simulink model "GA_PID_2DOF"  (R2024b)
settings: Solver=VariableStepDiscrete  StartTime=0.0  StopTime=40  RelTol=1e-3
values from neighbouring files (symbols this model uses):
  Kd1 = par(bestchrom, 3)    [GA_PID_Main.m]    (also in main_GA.m = par(pop_index, 3))
  Kd2 = par(bestchrom, 6)    [GA_PID_Main.m]    (also in main_GA.m = par(pop_index, 6))
  Ki1 = par(bestchrom, 2)    [GA_PID_Main.m]    (also in main_GA.m = par(pop_index, 2))
  Ki2 = par(bestchrom, 5)    [GA_PID_Main.m]    (also in main_GA.m = par(pop_index, 5))
  Kp1 = par(bestchrom, 1)    [GA_PID_Main.m]    (also in main_GA.m = par(bestchorm, 1), Ki1 = par(bestchorm, 2), Kd1 = par(bestch)
  Kp2 = par(bestchrom, 4)    [GA_PID_Main.m]    (also in main_GA.m = par(bestchorm, 4), Ki2 = par(bestchorm, 5), Kd2 = par(bestch)
settings Model: SimulationMode=accelerator  Creator=ENVY  LastModifiedBy=ENVY
settings DataIOCC: ReturnWorkspaceOutputs=off

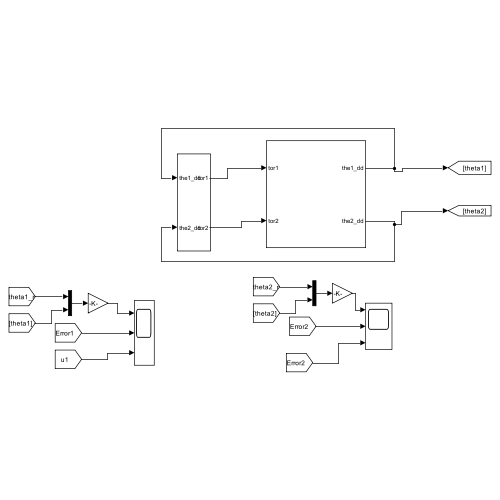
[thumbnail: Simulink's stored preview of the top-level diagram]
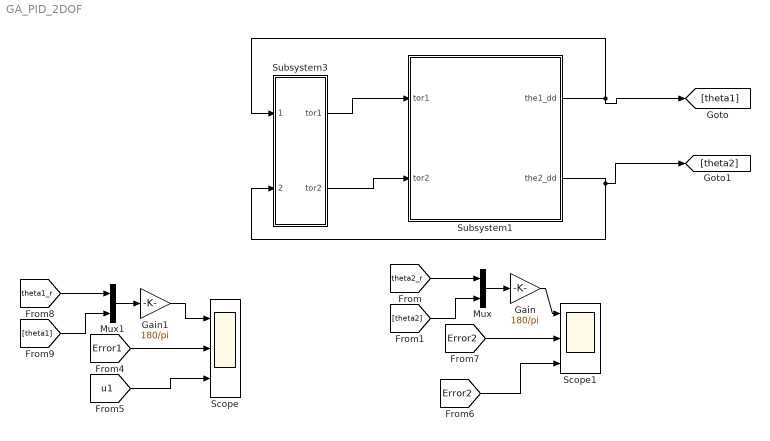
== system GA_PID_2DOF ==
  Gain : Gain  Gain=180/pi
  Gain1 : Gain  Gain=180/pi
  Mux : Mux  Inputs=2
  Mux1 : Mux  Inputs=2
  Scope : Scope  NumInputPorts=3
  Scope1 : Scope  NumInputPorts=3
  Subsystem1 : Subsystem
  Subsystem3 : Subsystem
  wires:
  Subsystem1/1(the1_dd) -> [theta1], Subsystem3/1(the1_dd)
  Subsystem1/2(the2_dd) -> Subsystem3/2(the2_dd), [theta2]
  Subsystem3/1(tor1) -> Subsystem1/1(tor1)
  Subsystem3/2(tor2) -> Subsystem1/2(tor2)
  [theta2_r] -> Mux/1
  [theta2] -> Mux/2
  Mux/1 -> Gain/1
  [theta1] -> Mux1/2
  [theta1_r] -> Mux1/1
  Mux1/1 -> Gain1/1
  Gain1/1 -> Scope/1
  [Error1] -> Scope/2
  [u1] -> Scope/3
  [Error2] -> Scope1/2
  [Error2] -> Scope1/3
  Gain/1 -> Scope1/1

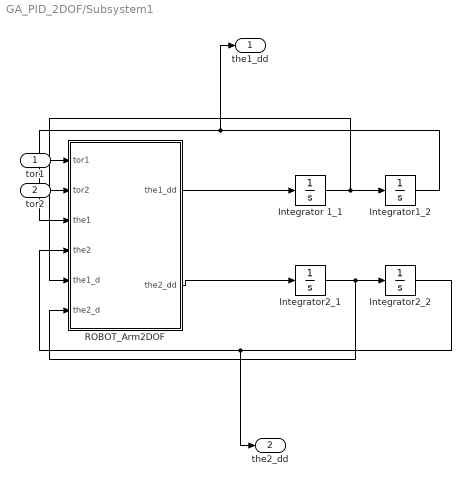
== system GA_PID_2DOF/Subsystem1 ==
  tor1 : Inport
  tor2 : Inport  Port=2
  Integrator 1_1 : Integrator
  Integrator1_2 : Integrator
  Integrator2_1 : Integrator
  Integrator2_2 : Integrator
  ROBOT_Arm2DOF : MATLAB Function  TreatAsAtomicUnit=on
  the1_dd : Outport
  the2_dd : Outport  Port=2
  wires:
  Integrator1_2/1 -> the1_dd/1, ROBOT_Arm2DOF/3(the1)
  ROBOT_Arm2DOF/1(the1_dd) -> Integrator 1_1/1
  tor2/1 -> ROBOT_Arm2DOF/2(tor2)
  Integrator2_2/1 -> the2_dd/1, ROBOT_Arm2DOF/4(the2)
  Integrator2_1/1 -> ROBOT_Arm2DOF/6(the2_d), Integrator2_2/1
  tor1/1 -> ROBOT_Arm2DOF/1(tor1)
  Integrator 1_1/1 -> ROBOT_Arm2DOF/5(the1_d), Integrator1_2/1
  ROBOT_Arm2DOF/2(the2_dd) -> Integrator2_1/1

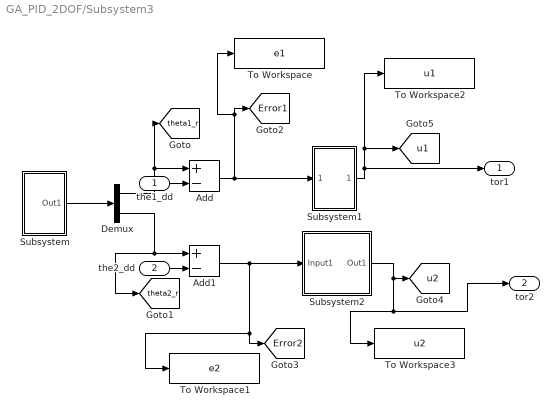
== system GA_PID_2DOF/Subsystem3 ==
  the1_dd : Inport
  the2_dd : Inport  Port=2
  Add : Sum  Inputs=+-
  Add1 : Sum  Inputs=+-
  Demux : Demux  Outputs=2
  Subsystem : Subsystem
  Subsystem1 : Subsystem
  Subsystem2 : Subsystem
  To Workspace : ToWorkspace  VariableName=e1  SampleTime=-1
  To Workspace1 : ToWorkspace  VariableName=e2  SampleTime=-1
  To Workspace2 : ToWorkspace  VariableName=u1  SampleTime=-1
  To Workspace3 : ToWorkspace  VariableName=u2  SampleTime=-1
  tor1 : Outport
  tor2 : Outport  Port=2
  tag scope: Error1=global, Error2=global, theta1_r=global, theta2_r=global, u1=global, u2=global
  wires:
  Demux/2 -> [theta2_r], Add1/1
  Add1/1 -> To Workspace1/1, [Error2], Subsystem2/1(Input1)
  Subsystem/1(Out1) -> Demux/1
  Add/1 -> To Workspace/1, [Error1], Subsystem1/1(Input)
  the1_dd/1 -> Add/2
  Demux/1 -> [theta1_r], Add/1
  Subsystem2/1(Out1) -> To Workspace3/1, tor2/1, [u2]
  Subsystem1/1(Out1) -> tor1/1, [u1], To Workspace2/1
  the2_dd/1 -> Add1/2

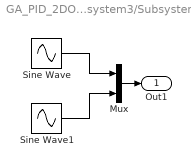
== system GA_PID_2DOF/Subsystem3/Subsystem ==
  Mux : Mux  Inputs=2
  Sine Wave : Sin  Amplitude=pi/6  Frequency=2*pi*0.1  SampleTime=0.01
  Sine Wave1 : Sin  Amplitude=pi/6  Frequency=2*pi*0.1  Phase=pi/6  SampleTime=0.01
  Out1 : Outport
  wires:
  Sine Wave1/1 -> Mux/2
  Sine Wave/1 -> Mux/1
  Mux/1 -> Out1/1

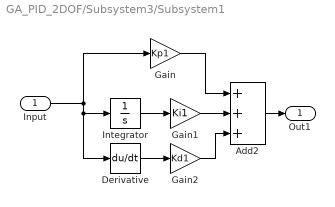
== system GA_PID_2DOF/Subsystem3/Subsystem1 ==
  Input : Inport
  Add2 : Sum  Inputs=+++
  Derivative : Derivative
  Gain : Gain  Gain=Kp1
  Gain1 : Gain  Gain=Ki1
  Gain2 : Gain  Gain=Kd1
  Integrator : Integrator
  Out1 : Outport
  wires:
  Gain2/1 -> Add2/3
  Input/1 -> Integrator/1, Derivative/1, Gain/1
  Derivative/1 -> Gain2/1
  Add2/1 -> Out1/1
  Gain/1 -> Add2/1
  Integrator/1 -> Gain1/1
  Gain1/1 -> Add2/2

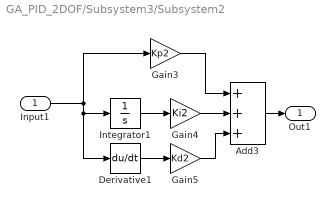
== system GA_PID_2DOF/Subsystem3/Subsystem2 ==
  Input1 : Inport
  Add3 : Sum  Inputs=+++
  Derivative1 : Derivative
  Gain3 : Gain  Gain=Kp2
  Gain4 : Gain  Gain=Ki2
  Gain5 : Gain  Gain=Kd2
  Integrator1 : Integrator
  Out1 : Outport
  wires:
  Gain5/1 -> Add3/3
  Gain3/1 -> Add3/1
  Input1/1 -> Integrator1/1, Derivative1/1, Gain3/1
  Add3/1 -> Out1/1
  Gain4/1 -> Add3/2
  Derivative1/1 -> Gain5/1
  Integrator1/1 -> Gain4/1

== matlab function GA_PID_2DOF/Subsystem1/ROBOT_Arm2DOF ==
  data: tor1 input; the1_dd output; tor2 input; the1 input; the2 input; the1_d input; the2_d input; the2_dd output
function [the1_dd, the2_dd] = fcn(tor1, tor2, the1, the2, the1_d, the2_d)
%#codegen
% Modèle dynamique du bras robotique 2-DoF
% Entrées: torques (Nm), positions (rad), vitesses (rad/s)
% Sorties: accélérations (rad/s²)

% --- Paramètres physiques ---
J1 = 0.05;      % Moment d'inertie joint 1 [kg·m²]
J2 = 0.05;      % Moment d'inertie joint 2 [kg·m²]
m1 = 1.0;       % Masse lien 1 [kg]
m2 = 1.0;       % Masse lien 2 [kg]
l1 = 1.0;       % Longueur lien 1 [m]
l2 = 1.0;       % Longueur lien 2 [m]
lc1 = 0.4;      % Distance CG lien 1 [m]
lc2 = 0.4;      % Distance CG lien 2 [m]
g = 9.81;       % Gravité [m/s²]

% --- Calculs intermédiaires ---
c2 = cos(the2);   % cos(theta2)
s2 = sin(the2);   % sin(theta2)
c12 = cos(the1 + the2);  % cos(theta1 + theta2)

% --- Matrice d'inertie M(theta) ---
% Élément M11
M11 = J1 + J2 + m1*lc1^2 + m2*(l1^2 + lc2^2 + 2*l1*lc2*c2);

% Élément M12 = M21
M12 = J2 + m2*(lc2^2 + l1*lc2*c2);

% Élément M22
M22 = J2 + m2*lc2^2;

% Construction de la matrice M
M = [M11, M12;
     M12, M22];  % Car M21 = M12 (matrice symétrique)

% --- Matrice de Coriolis/Centrifuge C(theta, theta_dot) ---
% Terme -m2*l1*lc2*s2
h = -m2*l1*lc2*s2;

% Construction de la matrice C
% Note: C est une matrice 2x2 selon la formule du manuel
C = [h*the2_d,     h*(the1_d + the2_d);
     -h*the1_d,    0];

% --- Vecteur de gravité G(theta) ---
G1 = (m1 + m2)*g*lc1*cos(the1) + m2*g*lc2*c12;
G2 = m2*g*lc2*c12;

G = [G1; G2];

% --- Vecteur d'état (vitesses) ---
theta_dot = [the1_d; the2_d];

% --- Calcul de l'accélération ---
% Équation: M * theta_ddot = tau - C * theta_dot - G
% Donc: theta_ddot = inv(M) * (tau - C*theta_dot - G)

tau = [tor1; tor2];  % Vecteur de couples

% Calcul du terme droit de l'équation
right_side = tau - C*theta_dot - G;

% Résolution pour theta_ddot (accélérations)
% Utilisation de l'opérateur backslash (plus stable que inv(M))
theta_ddot = M \ right_side;

% --- Extraction des sorties ---
the1_dd = theta_ddot(1);
the2_dd = theta_ddot(2);

end
